simulink model "sig_kadet"  (R2022a)
settings: Solver=FixedStepAuto  StartTime=0.0  StopTime=10.0  FixedStep=framePeriod_s  RelTol=1e-3
undefined symbols (not defined in the file): Control, DiscIntNeverNeededParam, framePeriod_s
libraries: slpidlib x10, aerolibconvert2 x7, simulink_extras x2
(part 2 of 2)

== system sig_kadet/Control Laws/Attitude Feedback/Pitch Controller ==
  note: Pitch damper
  note: Map stick to pitch angle command
  Pitch Stick : Inport
  Pitch Angle [rad] : Inport  Port=2
  Pitch Rate [rad/s] : Inport  Port=3
  Angle Conversion : aerolibconvert2/Angle Conversion  IU=deg  OU=rad
  Constant : Constant  Value=Control.Attitude.Pitch.ref_deg  OutDataTypeStr=single
  Constant1 : Constant  Value=Control.Attitude.Pitch.d  OutDataTypeStr=single
  Constant2 : Constant  Value=framePeriod_s  OutDataTypeStr=single
  PID Controller : slpidlib/PID Controller  Controller=PID  Form=Parallel  TimeDomain=Discrete-time  UseExternalTs=on  SampleTime=-1  IntegratorMethod=Forward Euler  FilterMethod=Forward Euler  ControllerParametersSource=internal  P=Control.Attitude.Pitch.p  I=Control.Attitude.Pitch.i  D=0  UseFilter=off  N=100  TunerSelectOption=Transfer Function Based (PID Tuner App)  ZeroCross=off  InitialConditionSource=internal  InitialConditionForIntegrator=0  InitialConditionForFilter=0  DifferentiatorICPrevScaledInput=0  ExternalReset=none  TrackingMode=off  Kt=1  LimitOutput=on  SatLimitsSource=internal  UpperSaturationLimit=deg2rad(Control.elev_lim_deg)  LowerSaturationLimit=-deg2rad(Control.elev_lim_deg)  LinearizeAsGain=on  AntiWindupMode=clamping  Kb=1  PGainOutDataTypeStr=single  PProdOutDataTypeStr=single  POutMin=[]  POutMax=[]  IGainOutDataTypeStr=single  IProdOutDataTypeStr=single  IOutMin=[]  IOutMax=[]  DGainOutDataTypeStr=single  DProdOutDataTypeStr=single  DOutMin=[]  DOutMax=[]  NOutMin=[]  NOutMax=[]  SumOutDataTypeStr=single  SumOutMin=[]  SumOutMax=[]  SaturationOutDataTypeStr=single  SaturationOutMin=[]  SaturationOutMax=[]  PParamMin=[]  PParamMax=[]  IParamMin=[]  IParamMax=[]  DParamMin=[]  DParamMax=[]  NParamMin=[]  NParamMax=[]  KbParamMin=[]  KbParamMax=[]  KtParamMin=[]  KtParamMax=[]  KbOutMin=[]  KbOutMax=[]  KtOutMin=[]  KtOutMax=[]  IntegratorOutMin=[]  IntegratorOutMax=[]  FilterOutMin=[]  FilterOutMax=[]  SumI1OutMin=[]  SumI1OutMax=[]  SumI2OutMin=[]  SumI2OutMax=[]  SumI3OutMin=[]  SumI3OutMax=[]  SumI4OutMin=[]  SumI4OutMax=[]  SumDOutMin=[]  SumDOutMax=[]  DifferentiatorOutMin=[]  DifferentiatorOutMax=[]  FilterDiffOutCoefMin=[]  FilterDiffOutCoefMax=[]  ReciprocalOutMin=[]  ReciprocalOutMax=[]  SumDenOutMin=[]  SumDenOutMax=[]  SumNumOutMin=[]  SumNumOutMax=[]  DivideOutMin=[]  DivideOutMax=[]  UdiffTsProdOutMin=[]  UdiffTsProdOutMax=[]  NTsProdOutMin=[]  NTsProdOutMax=[]  UintegralTsProdOutMin=[]  UintegralTsProdOutMax=[]  UngainTsProdOutMin=[]  UngainTsProdOutMax=[]  IntegratorContinuousStateAttributes=''  IntegratorStateMustResolveToSignalObject=off  IntegratorRTWStateStorageClass=Auto  FilterContinuousStateAttributes=''  FilterStateMustResolveToSignalObject=off  FilterRTWStateStorageClass=Auto  ParallelPVariant=InternalParameters  IdealPVariant=Disabled  IVariant=InternalParameters  DVariant=InternalParameters  IntegratorVariant=Discrete  SatVariant=Enabled  AWVariant=DiscClampingParallel  PCopyVariant=Disabled  TRVariant=Disabled  FdbkBlocksVariant=Forward  IdealPFdbkVariant=Disabled  SatFdbkVariant=Disabled  DerivativeFilterVariant=Differentiator  NVariant=Passthrough  NCopyVariant=Disabled_SignalSpec  FilterICVariant=InternalICsDifferentiator  IntegratorICVariant=InternalICs  ExternalResetVariant=Disabled  TRSumVariant=Passthrough  SumFdbkVariant=Disabled  SumVariant=Sum_PID  TsampFilterVariant=ExternalTs  TsampNgainVariant=Passthrough  TsampIntegralVariant=ExternalTs  ExternalSaturationOutDataTypeStr=Inherit: Same as second input
  Product : Product  OutDataTypeStr=single
  Product1 : Product
  Subtract : Sum  Inputs=+-
  Subtract1 : Sum  Inputs=+-
  Elevator Cmd [rad] : Outport
  wires:
  Pitch Stick/1 -> Product/2
  Constant/1 -> Product/1
  Product/1 -> Angle Conversion/1
  Angle Conversion/1 -> Subtract/1
  Pitch Angle [rad]/1 -> Subtract/2
  PID Controller/1 -> Subtract1/1
  Product1/1 -> Subtract1/2
  Pitch Rate [rad/s]/1 -> Product1/1
  Constant1/1 -> Product1/2
  Subtract1/1 -> Elevator Cmd [rad]/1
  Constant2/1 -> PID Controller/2
  Subtract/1 -> PID Controller/1

== system sig_kadet/Control Laws/Attitude Feedback/Roll Controller ==
  note: Map stick to roll angle command
  note: Roll damper
  Roll Stick : Inport
  Roll Angle [rad] : Inport  Port=2
  Roll Rate [rad/s] : Inport  Port=3
  Angle Conversion : aerolibconvert2/Angle Conversion  IU=deg  OU=rad
  Constant : Constant  Value=Control.Attitude.Roll.ref_deg  OutDataTypeStr=single
  Constant1 : Constant  Value=Control.Attitude.Roll.d  OutDataTypeStr=single
  Constant2 : Constant  Value=framePeriod_s  OutDataTypeStr=single
  PID Controller : slpidlib/PID Controller  Controller=PID  Form=Parallel  TimeDomain=Discrete-time  UseExternalTs=on  SampleTime=-1  IntegratorMethod=Forward Euler  FilterMethod=Forward Euler  ControllerParametersSource=internal  P=Control.Attitude.Roll.p  I=Control.Attitude.Roll.i  D=0  UseFilter=off  N=100  TunerSelectOption=Transfer Function Based (PID Tuner App)  ZeroCross=off  InitialConditionSource=internal  InitialConditionForIntegrator=0  InitialConditionForFilter=0  DifferentiatorICPrevScaledInput=0  ExternalReset=none  TrackingMode=off  Kt=1  LimitOutput=on  SatLimitsSource=internal  UpperSaturationLimit=deg2rad(Control.ail_lim_deg)  LowerSaturationLimit=-deg2rad(Control.ail_lim_deg)  LinearizeAsGain=on  AntiWindupMode=clamping  Kb=1  PGainOutDataTypeStr=single  PProdOutDataTypeStr=single  POutMin=[]  POutMax=[]  IGainOutDataTypeStr=single  IProdOutDataTypeStr=single  IOutMin=[]  IOutMax=[]  DGainOutDataTypeStr=single  DProdOutDataTypeStr=single  DOutMin=[]  DOutMax=[]  NOutMin=[]  NOutMax=[]  SumOutDataTypeStr=single  SumOutMin=[]  SumOutMax=[]  SaturationOutDataTypeStr=single  SaturationOutMin=[]  SaturationOutMax=[]  PParamMin=[]  PParamMax=[]  IParamMin=[]  IParamMax=[]  DParamMin=[]  DParamMax=[]  NParamMin=[]  NParamMax=[]  KbParamMin=[]  KbParamMax=[]  KtParamMin=[]  KtParamMax=[]  KbOutMin=[]  KbOutMax=[]  KtOutMin=[]  KtOutMax=[]  IntegratorOutMin=[]  IntegratorOutMax=[]  FilterOutMin=[]  FilterOutMax=[]  SumI1OutMin=[]  SumI1OutMax=[]  SumI2OutMin=[]  SumI2OutMax=[]  SumI3OutMin=[]  SumI3OutMax=[]  SumI4OutMin=[]  SumI4OutMax=[]  SumDOutMin=[]  SumDOutMax=[]  DifferentiatorOutMin=[]  DifferentiatorOutMax=[]  FilterDiffOutCoefMin=[]  FilterDiffOutCoefMax=[]  ReciprocalOutMin=[]  ReciprocalOutMax=[]  SumDenOutMin=[]  SumDenOutMax=[]  SumNumOutMin=[]  SumNumOutMax=[]  DivideOutMin=[]  DivideOutMax=[]  UdiffTsProdOutMin=[]  UdiffTsProdOutMax=[]  NTsProdOutMin=[]  NTsProdOutMax=[]  UintegralTsProdOutMin=[]  UintegralTsProdOutMax=[]  UngainTsProdOutMin=[]  UngainTsProdOutMax=[]  IntegratorContinuousStateAttributes=''  IntegratorStateMustResolveToSignalObject=off  IntegratorRTWStateStorageClass=Auto  FilterContinuousStateAttributes=''  FilterStateMustResolveToSignalObject=off  FilterRTWStateStorageClass=Auto  ParallelPVariant=InternalParameters  IdealPVariant=Disabled  IVariant=InternalParameters  DVariant=InternalParameters  IntegratorVariant=Discrete  SatVariant=Enabled  AWVariant=DiscClampingParallel  PCopyVariant=Disabled  TRVariant=Disabled  FdbkBlocksVariant=Forward  IdealPFdbkVariant=Disabled  SatFdbkVariant=Disabled  DerivativeFilterVariant=Differentiator  NVariant=Passthrough  NCopyVariant=Disabled_SignalSpec  FilterICVariant=InternalICsDifferentiator  IntegratorICVariant=InternalICs  ExternalResetVariant=Disabled  TRSumVariant=Passthrough  SumFdbkVariant=Disabled  SumVariant=Sum_PID  TsampFilterVariant=ExternalTs  TsampNgainVariant=Passthrough  TsampIntegralVariant=ExternalTs  ExternalSaturationOutDataTypeStr=Inherit: Same as second input
  Product : Product  OutDataTypeStr=single
  Product1 : Product
  Subtract : Sum  Inputs=+-
  Subtract1 : Sum  Inputs=+-
  Aileron Cmd [rad] : Outport
  wires:
  Constant2/1 -> PID Controller/2
  Subtract1/1 -> Aileron Cmd [rad]/1
  Constant1/1 -> Product1/2
  Roll Rate [rad/s]/1 -> Product1/1
  Product1/1 -> Subtract1/2
  PID Controller/1 -> Subtract1/1
  Subtract/1 -> PID Controller/1
  Roll Angle [rad]/1 -> Subtract/2
  Angle Conversion/1 -> Subtract/1
  Product/1 -> Angle Conversion/1
  Constant/1 -> Product/1
  Roll Stick/1 -> Product/2

== system sig_kadet/Control Laws/Attitude Feedback/Yaw Damper ==
  Yaw Rate [rad/s] : Inport
  Discrete Transfer Fcn : DiscreteTransferFcn  Numerator=[-0.065 0.065]  Denominator=[1 -0.9608]
  Rudder Cmd [rad] : Outport
  wires:
  Discrete Transfer Fcn/1 -> Rudder Cmd [rad]/1
  Yaw Rate [rad/s]/1 -> Discrete Transfer Fcn/1

== system sig_kadet/Control Laws/Autopilot/Geschwindigkeitsregler ==
  note: desired airspeed for current waypoint
  Vehicle States : Inport
  Telemetry Data : Inport  Port=2
  Bus Selector : BusSelector  OutputSignals=ias_mps
  Bus Selector1 : BusSelector  OutputSignals=param1
  Bus Selector2 : BusSelector  OutputSignals=flight_plan,current_waypoint
  PID Controller : slpidlib/PID Controller  Controller=PID  Form=Parallel  TimeDomain=Discrete-time  UseExternalTs=on  SampleTime=-1  IntegratorMethod=Forward Euler  FilterMethod=Forward Euler  ControllerParametersSource=internal  P=1  I=1  D=0  UseFilter=off  N=100  TunerSelectOption=Transfer Function Based (PID Tuner App)  InitialConditionSource=internal  InitialConditionForIntegrator=0  InitialConditionForFilter=0  DifferentiatorICPrevScaledInput=0  ExternalReset=none  TrackingMode=off  Kt=1  LimitOutput=off  SatLimitsSource=internal  UpperSaturationLimit=inf  LowerSaturationLimit=-inf  LinearizeAsGain=on  AntiWindupMode=none  Kb=1  POutMin=[]  POutMax=[]  IOutMin=[]  IOutMax=[]  DOutMin=[]  DOutMax=[]  NOutMin=[]  NOutMax=[]  SumOutMin=[]  SumOutMax=[]  SaturationOutMin=[]  SaturationOutMax=[]  PParamMin=[]  PParamMax=[]  IParamMin=[]  IParamMax=[]  DParamMin=[]  DParamMax=[]  NParamMin=[]  NParamMax=[]  KbParamMin=[]  KbParamMax=[]  KtParamMin=[]  KtParamMax=[]  KbOutMin=[]  KbOutMax=[]  KtOutMin=[]  KtOutMax=[]  IntegratorOutMin=[]  IntegratorOutMax=[]  FilterOutMin=[]  FilterOutMax=[]  SumI1OutMin=[]  SumI1OutMax=[]  SumI2OutMin=[]  SumI2OutMax=[]  SumI3OutMin=[]  SumI3OutMax=[]  SumI4OutMin=[]  SumI4OutMax=[]  SumDOutMin=[]  SumDOutMax=[]  DifferentiatorOutMin=[]  DifferentiatorOutMax=[]  FilterDiffOutCoefMin=[]  FilterDiffOutCoefMax=[]  ReciprocalOutMin=[]  ReciprocalOutMax=[]  SumDenOutMin=[]  SumDenOutMax=[]  SumNumOutMin=[]  SumNumOutMax=[]  DivideOutMin=[]  DivideOutMax=[]  UdiffTsProdOutMin=[]  UdiffTsProdOutMax=[]  NTsProdOutMin=[]  NTsProdOutMax=[]  UintegralTsProdOutMin=[]  UintegralTsProdOutMax=[]  UngainTsProdOutMin=[]  UngainTsProdOutMax=[]  IntegratorContinuousStateAttributes=''  IntegratorStateMustResolveToSignalObject=off  IntegratorRTWStateStorageClass=Auto  FilterContinuousStateAttributes=''  FilterStateMustResolveToSignalObject=off  FilterRTWStateStorageClass=Auto  ParallelPVariant=InternalParameters  IdealPVariant=Disabled  IVariant=InternalParameters  DVariant=InternalParameters  IntegratorVariant=Discrete  SatVariant=Disabled  AWVariant=Passthrough  PCopyVariant=Disabled  TRVariant=Disabled  FdbkBlocksVariant=Forward  IdealPFdbkVariant=Disabled  SatFdbkVariant=Disabled  DerivativeFilterVariant=Differentiator  NVariant=Passthrough  NCopyVariant=Disabled_SignalSpec  FilterICVariant=InternalICsDifferentiator  IntegratorICVariant=InternalICs  ExternalResetVariant=Disabled  TRSumVariant=Passthrough  SumFdbkVariant=Disabled  SumVariant=Sum_PID  TsampFilterVariant=ExternalTs  TsampNgainVariant=Passthrough  TsampIntegralVariant=ExternalTs  ExternalSaturationOutDataTypeStr=Inherit: Same as second input
  Selector : Selector  IndexMode=Zero-based  InputPortWidth=500  IndexOptions=Index vector (port)  Indices=[1 3]  OutputSizes=1
  Sum : Sum  Inputs=|+-
  Throttle [0-1] : Outport
  wires:
  Vehicle States/1 -> Bus Selector/1
  Bus Selector/1 -> Sum/2  "<ias_mps>"
  Telemetry Data/1 -> Bus Selector2/1
  Bus Selector2/1 -> Selector/1  "<flight_plan>"
  Selector/1 -> Bus Selector1/1  "current waypoint parameter"
  Bus Selector2/2 -> Selector/2  "<current_waypoint>"
  Bus Selector1/1 -> Sum/1  "<param1>"
  Sum/1 -> PID Controller/1  "airspeed error [m/s]"
  PID Controller/1 -> Throttle [0-1]/1  "Throttle [0-1]"

== system sig_kadet/Control Laws/Autopilot/Gierdämpfer ==
  Vehicle States : Inport
  Bus Selector : BusSelector  OutputSignals=gyro_radps
  Demux : Demux  Outputs=3
  Discrete Transfer Fcn : DiscreteTransferFcn  Denominator=[1 6]
  Gain : Gain
  Terminator : Terminator
  Terminator1 : Terminator
  Out1 : Outport
  wires:
  Vehicle States/1 -> Bus Selector/1
  Bus Selector/1 -> Demux/1  "<gyro_radps>"
  Demux/1 -> Terminator/1  "p [rad/s]"
  Demux/2 -> Terminator1/1  "q [rad/s]"
  Demux/3 -> Gain/1  "r [rad/s]"
  Gain/1 -> Discrete Transfer Fcn/1

== system sig_kadet/Control Laws/Autopilot/Headingregler ==
  x aircraft [m] : Inport
  y aircraft [m] : Inport  Port=2
  x waypoint [m] : Inport  Port=3
  y waypoint [m] : Inport  Port=4
  Vehicle States : Inport  Port=5
  Bus Selector : BusSelector  OutputSignals=heading_rad
  MATLAB Function : MATLAB Function  TreatAsAtomicUnit=on
  PID Controller : slpidlib/PID Controller  Controller=PID  Form=Parallel  TimeDomain=Discrete-time  UseExternalTs=on  SampleTime=-1  IntegratorMethod=Forward Euler  FilterMethod=Forward Euler  ControllerParametersSource=internal  P=1  I=0  D=0  UseFilter=off  N=100  TunerSelectOption=Transfer Function Based (PID Tuner App)  InitialConditionSource=internal  InitialConditionForIntegrator=0  InitialConditionForFilter=0  DifferentiatorICPrevScaledInput=0  ExternalReset=none  TrackingMode=off  Kt=1  LimitOutput=off  SatLimitsSource=internal  UpperSaturationLimit=inf  LowerSaturationLimit=-inf  LinearizeAsGain=on  AntiWindupMode=none  Kb=1  POutMin=[]  POutMax=[]  IOutMin=[]  IOutMax=[]  DOutMin=[]  DOutMax=[]  NOutMin=[]  NOutMax=[]  SumOutMin=[]  SumOutMax=[]  SaturationOutMin=[]  SaturationOutMax=[]  PParamMin=[]  PParamMax=[]  IParamMin=[]  IParamMax=[]  DParamMin=[]  DParamMax=[]  NParamMin=[]  NParamMax=[]  KbParamMin=[]  KbParamMax=[]  KtParamMin=[]  KtParamMax=[]  KbOutMin=[]  KbOutMax=[]  KtOutMin=[]  KtOutMax=[]  IntegratorOutMin=[]  IntegratorOutMax=[]  FilterOutMin=[]  FilterOutMax=[]  SumI1OutMin=[]  SumI1OutMax=[]  SumI2OutMin=[]  SumI2OutMax=[]  SumI3OutMin=[]  SumI3OutMax=[]  SumI4OutMin=[]  SumI4OutMax=[]  SumDOutMin=[]  SumDOutMax=[]  DifferentiatorOutMin=[]  DifferentiatorOutMax=[]  FilterDiffOutCoefMin=[]  FilterDiffOutCoefMax=[]  ReciprocalOutMin=[]  ReciprocalOutMax=[]  SumDenOutMin=[]  SumDenOutMax=[]  SumNumOutMin=[]  SumNumOutMax=[]  DivideOutMin=[]  DivideOutMax=[]  UdiffTsProdOutMin=[]  UdiffTsProdOutMax=[]  NTsProdOutMin=[]  NTsProdOutMax=[]  UintegralTsProdOutMin=[]  UintegralTsProdOutMax=[]  UngainTsProdOutMin=[]  UngainTsProdOutMax=[]  IntegratorContinuousStateAttributes=''  IntegratorStateMustResolveToSignalObject=off  IntegratorRTWStateStorageClass=Auto  FilterContinuousStateAttributes=''  FilterStateMustResolveToSignalObject=off  FilterRTWStateStorageClass=Auto  ParallelPVariant=InternalParameters  IdealPVariant=Disabled  IVariant=InternalParameters  DVariant=InternalParameters  IntegratorVariant=Discrete  SatVariant=Disabled  AWVariant=Passthrough  PCopyVariant=Disabled  TRVariant=Disabled  FdbkBlocksVariant=Forward  IdealPFdbkVariant=Disabled  SatFdbkVariant=Disabled  DerivativeFilterVariant=Differentiator  NVariant=Passthrough  NCopyVariant=Disabled_SignalSpec  FilterICVariant=InternalICsDifferentiator  IntegratorICVariant=InternalICs  ExternalResetVariant=Disabled  TRSumVariant=Passthrough  SumFdbkVariant=Disabled  SumVariant=Sum_PID  TsampFilterVariant=ExternalTs  TsampNgainVariant=Passthrough  TsampIntegralVariant=ExternalTs  ExternalSaturationOutDataTypeStr=Inherit: Same as second input
  aileronausschlag : Outport
  heading error : Outport  Port=2
  wires:
  x aircraft [m]/1 -> MATLAB Function/1(x_ac)
  y aircraft [m]/1 -> MATLAB Function/2(y_ac)
  x waypoint [m]/1 -> MATLAB Function/3(x_wp)
  y waypoint [m]/1 -> MATLAB Function/4(y_wp)
  Vehicle States/1 -> Bus Selector/1
  Bus Selector/1 -> MATLAB Function/5(heading)  "<heading_rad>"
  MATLAB Function/1(heading_error) -> heading error/1, PID Controller/1
  PID Controller/1 -> aileronausschlag/1  "aileron ausschlag"

== system sig_kadet/Control Laws/Autopilot/Höhenregler ==
  z_aircraft [m] : Inport
  z_waypoint [m] : Inport  Port=2
  Vehicel States : Inport  Port=3
  Bus Selector : BusSelector  OutputSignals=pitch_rad,gyro_radps
  Demux : Demux  Outputs=3
  PID Controller : slpidlib/PID Controller  Controller=PID  Form=Parallel  TimeDomain=Discrete-time  UseExternalTs=on  SampleTime=-1  IntegratorMethod=Forward Euler  FilterMethod=Forward Euler  ControllerParametersSource=internal  P=1  I=1  D=0  UseFilter=off  N=100  TunerSelectOption=Transfer Function Based (PID Tuner App)  InitialConditionSource=internal  InitialConditionForIntegrator=0  InitialConditionForFilter=0  DifferentiatorICPrevScaledInput=0  ExternalReset=none  TrackingMode=off  Kt=1  LimitOutput=off  SatLimitsSource=internal  UpperSaturationLimit=inf  LowerSaturationLimit=-inf  LinearizeAsGain=on  AntiWindupMode=none  Kb=1  POutMin=[]  POutMax=[]  IOutMin=[]  IOutMax=[]  DOutMin=[]  DOutMax=[]  NOutMin=[]  NOutMax=[]  SumOutMin=[]  SumOutMax=[]  SaturationOutMin=[]  SaturationOutMax=[]  PParamMin=[]  PParamMax=[]  IParamMin=[]  IParamMax=[]  DParamMin=[]  DParamMax=[]  NParamMin=[]  NParamMax=[]  KbParamMin=[]  KbParamMax=[]  KtParamMin=[]  KtParamMax=[]  KbOutMin=[]  KbOutMax=[]  KtOutMin=[]  KtOutMax=[]  IntegratorOutMin=[]  IntegratorOutMax=[]  FilterOutMin=[]  FilterOutMax=[]  SumI1OutMin=[]  SumI1OutMax=[]  SumI2OutMin=[]  SumI2OutMax=[]  SumI3OutMin=[]  SumI3OutMax=[]  SumI4OutMin=[]  SumI4OutMax=[]  SumDOutMin=[]  SumDOutMax=[]  DifferentiatorOutMin=[]  DifferentiatorOutMax=[]  FilterDiffOutCoefMin=[]  FilterDiffOutCoefMax=[]  ReciprocalOutMin=[]  ReciprocalOutMax=[]  SumDenOutMin=[]  SumDenOutMax=[]  SumNumOutMin=[]  SumNumOutMax=[]  DivideOutMin=[]  DivideOutMax=[]  UdiffTsProdOutMin=[]  UdiffTsProdOutMax=[]  NTsProdOutMin=[]  NTsProdOutMax=[]  UintegralTsProdOutMin=[]  UintegralTsProdOutMax=[]  UngainTsProdOutMin=[]  UngainTsProdOutMax=[]  IntegratorContinuousStateAttributes=''  IntegratorStateMustResolveToSignalObject=off  IntegratorRTWStateStorageClass=Auto  FilterContinuousStateAttributes=''  FilterStateMustResolveToSignalObject=off  FilterRTWStateStorageClass=Auto  ParallelPVariant=InternalParameters  IdealPVariant=Disabled  IVariant=InternalParameters  DVariant=InternalParameters  IntegratorVariant=Discrete  SatVariant=Disabled  AWVariant=Passthrough  PCopyVariant=Disabled  TRVariant=Disabled  FdbkBlocksVariant=Forward  IdealPFdbkVariant=Disabled  SatFdbkVariant=Disabled  DerivativeFilterVariant=Differentiator  NVariant=Passthrough  NCopyVariant=Disabled_SignalSpec  FilterICVariant=InternalICsDifferentiator  IntegratorICVariant=InternalICs  ExternalResetVariant=Disabled  TRSumVariant=Passthrough  SumFdbkVariant=Disabled  SumVariant=Sum_PID  TsampFilterVariant=ExternalTs  TsampNgainVariant=Passthrough  TsampIntegralVariant=ExternalTs  ExternalSaturationOutDataTypeStr=Inherit: Same as second input
  PID Controller1 : slpidlib/PID Controller  Controller=PID  Form=Parallel  TimeDomain=Discrete-time  UseExternalTs=on  SampleTime=-1  IntegratorMethod=Forward Euler  FilterMethod=Forward Euler  ControllerParametersSource=internal  P=1  I=1  D=0  UseFilter=off  N=100  TunerSelectOption=Transfer Function Based (PID Tuner App)  InitialConditionSource=internal  InitialConditionForIntegrator=0  InitialConditionForFilter=0  DifferentiatorICPrevScaledInput=0  ExternalReset=none  TrackingMode=off  Kt=1  LimitOutput=off  SatLimitsSource=internal  UpperSaturationLimit=inf  LowerSaturationLimit=-inf  LinearizeAsGain=on  AntiWindupMode=none  Kb=1  POutMin=[]  POutMax=[]  IOutMin=[]  IOutMax=[]  DOutMin=[]  DOutMax=[]  NOutMin=[]  NOutMax=[]  SumOutMin=[]  SumOutMax=[]  SaturationOutMin=[]  SaturationOutMax=[]  PParamMin=[]  PParamMax=[]  IParamMin=[]  IParamMax=[]  DParamMin=[]  DParamMax=[]  NParamMin=[]  NParamMax=[]  KbParamMin=[]  KbParamMax=[]  KtParamMin=[]  KtParamMax=[]  KbOutMin=[]  KbOutMax=[]  KtOutMin=[]  KtOutMax=[]  IntegratorOutMin=[]  IntegratorOutMax=[]  FilterOutMin=[]  FilterOutMax=[]  SumI1OutMin=[]  SumI1OutMax=[]  SumI2OutMin=[]  SumI2OutMax=[]  SumI3OutMin=[]  SumI3OutMax=[]  SumI4OutMin=[]  SumI4OutMax=[]  SumDOutMin=[]  SumDOutMax=[]  DifferentiatorOutMin=[]  DifferentiatorOutMax=[]  FilterDiffOutCoefMin=[]  FilterDiffOutCoefMax=[]  ReciprocalOutMin=[]  ReciprocalOutMax=[]  SumDenOutMin=[]  SumDenOutMax=[]  SumNumOutMin=[]  SumNumOutMax=[]  DivideOutMin=[]  DivideOutMax=[]  UdiffTsProdOutMin=[]  UdiffTsProdOutMax=[]  NTsProdOutMin=[]  NTsProdOutMax=[]  UintegralTsProdOutMin=[]  UintegralTsProdOutMax=[]  UngainTsProdOutMin=[]  UngainTsProdOutMax=[]  IntegratorContinuousStateAttributes=''  IntegratorStateMustResolveToSignalObject=off  IntegratorRTWStateStorageClass=Auto  FilterContinuousStateAttributes=''  FilterStateMustResolveToSignalObject=off  FilterRTWStateStorageClass=Auto  ParallelPVariant=InternalParameters  IdealPVariant=Disabled  IVariant=InternalParameters  DVariant=InternalParameters  IntegratorVariant=Discrete  SatVariant=Disabled  AWVariant=Passthrough  PCopyVariant=Disabled  TRVariant=Disabled  FdbkBlocksVariant=Forward  IdealPFdbkVariant=Disabled  SatFdbkVariant=Disabled  DerivativeFilterVariant=Differentiator  NVariant=Passthrough  NCopyVariant=Disabled_SignalSpec  FilterICVariant=InternalICsDifferentiator  IntegratorICVariant=InternalICs  ExternalResetVariant=Disabled  TRSumVariant=Passthrough  SumFdbkVariant=Disabled  SumVariant=Sum_PID  TsampFilterVariant=ExternalTs  TsampNgainVariant=Passthrough  TsampIntegralVariant=ExternalTs  ExternalSaturationOutDataTypeStr=Inherit: Same as second input
  Sum : Sum  Inputs=|+-
  Sum1 : Sum  Inputs=|+-
  Sum2 : Sum  Inputs=|+-
  Terminator : Terminator
  Terminator1 : Terminator
  pitchrate damping gain : Gain
  delta_eta [deg] : Outport
  wires:
  z_waypoint [m]/1 -> Sum/1
  z_aircraft [m]/1 -> Sum/2
  Sum/1 -> PID Controller/1  "delta_z [m]"
  Vehicel States/1 -> Bus Selector/1
  Bus Selector/1 -> Sum1/2  "<pitch_rad>"
  PID Controller/1 -> Sum1/1  "desired pitch angele to get to desired altitude [rad]"
  Sum1/1 -> PID Controller1/1  "pitch angel error [rad]"
  PID Controller1/1 -> Sum2/1  "desired elevator deflection to get to desired pitch angle [deg]"
  Bus Selector/2 -> Demux/1  "<gyro_radps>"
  Demux/1 -> Terminator/1  "p [rad/s]"
  Demux/2 -> pitchrate damping gain/1  "q [rad/s]"
  Demux/3 -> Terminator1/1  "r [rad/s]"
  pitchrate damping gain/1 -> Sum2/2
  Sum2/1 -> delta_eta [deg]/1  "elevator deflection [deg]"

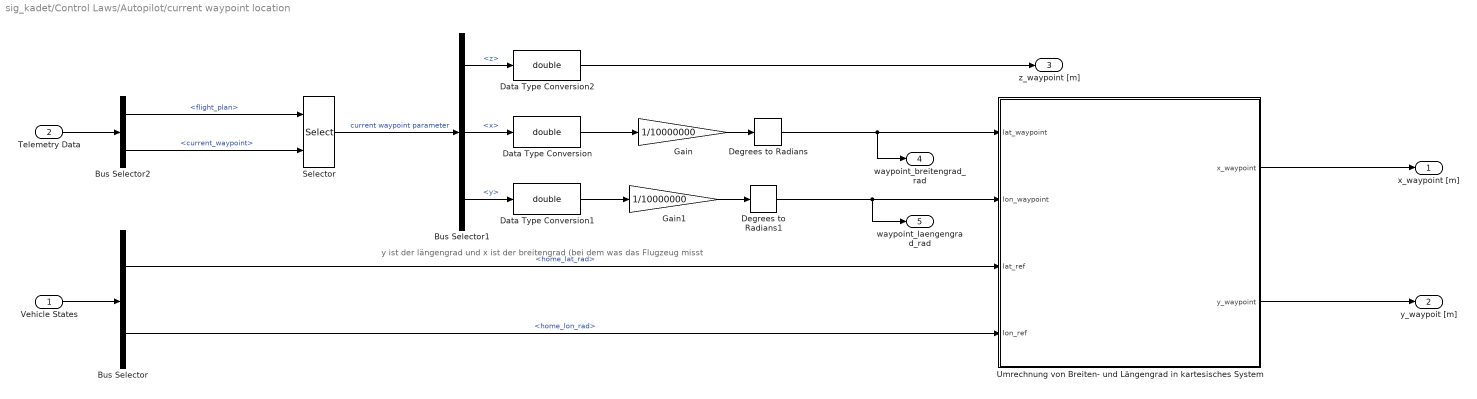
== system sig_kadet/Control Laws/Autopilot/current waypoint location ==
  note: y ist der längengrad und x ist der breitengrad (bei dem was das Flugzeug misst
  Vehicle States : Inport
  Telemetry Data : Inport  Port=2
  Bus Selector : BusSelector  OutputSignals=home_lat_rad,home_lon_rad
  Bus Selector1 : BusSelector  OutputSignals=z,x,y
  Bus Selector2 : BusSelector  OutputSignals=flight_plan,current_waypoint
  Data Type Conversion : DataTypeConversion  OutDataTypeStr=double  SaturateOnIntegerOverflow=off  RndMeth=Floor
  Data Type Conversion1 : DataTypeConversion  OutDataTypeStr=double  SaturateOnIntegerOverflow=off  RndMeth=Floor
  Data Type Conversion2 : DataTypeConversion  OutDataTypeStr=double  SaturateOnIntegerOverflow=off  RndMeth=Floor
  Degrees to Radians : simulink_extras/Transformations/Degrees to Radians
  Degrees to Radians1 : simulink_extras/Transformations/Degrees to Radians
  Gain : Gain  Gain=1/10000000
  Gain1 : Gain  Gain=1/10000000
  Selector : Selector  IndexMode=Zero-based  InputPortWidth=500  IndexOptions=Index vector (port)  Indices=[1 3]  OutputSizes=1
  Umrechnung von Breiten- und Längengrad in kartesisches System : MATLAB Function  TreatAsAtomicUnit=on
  x_waypoint [m] : Outport
  y_waypoit [m] : Outport  Port=2
  z_waypoint [m] : Outport  Port=3
  waypoint_breitengrad_rad : Outport  Port=4
  waypoint_laengengrad_rad : Outport  Port=5
  wires:
  Vehicle States/1 -> Bus Selector/1
  Telemetry Data/1 -> Bus Selector2/1
  Bus Selector2/1 -> Selector/1  "<flight_plan>"
  Bus Selector2/2 -> Selector/2  "<current_waypoint>"
  Selector/1 -> Bus Selector1/1  "current waypoint parameter"
  Bus Selector1/3 -> Data Type Conversion1/1  "<y>"
  Bus Selector1/2 -> Data Type Conversion/1  "<x>"
  Bus Selector1/1 -> Data Type Conversion2/1  "<z>"
  Bus Selector/1 -> Umrechnung von Breiten- und Längengrad in kartesisches System/3(lat_ref)  "<home_lat_rad>"
  Bus Selector/2 -> Umrechnung von Breiten- und Längengrad in kartesisches System/4(lon_ref)  "<home_lon_rad>"
  Umrechnung von Breiten- und Längengrad in kartesisches System/1(x_waypoint) -> x_waypoint [m]/1
  Umrechnung von Breiten- und Längengrad in kartesisches System/2(y_waypoint) -> y_waypoit [m]/1
  Data Type Conversion/1 -> Gain/1
  Data Type Conversion1/1 -> Gain1/1
  Data Type Conversion2/1 -> z_waypoint [m]/1
  Gain/1 -> Degrees to Radians/1
  Degrees to Radians/1 -> Umrechnung von Breiten- und Längengrad in kartesisches System/1(lat_waypoint), waypoint_breitengrad_rad/1
  Gain1/1 -> Degrees to Radians1/1
  Degrees to Radians1/1 -> Umrechnung von Breiten- und Längengrad in kartesisches System/2(lon_waypoint), waypoint_laengengrad_rad/1

== system sig_kadet/Control Laws/Autopilot/plane location ==
  Vehicle States : Inport
  Bus Selector : BusSelector  OutputSignals=lat_rad,lon_rad,home_lat_rad,home_lon_rad,alt_msl_m
  Umrechnung von Breiten- und Längengrad in kartesisches System : MATLAB Function  TreatAsAtomicUnit=on
  x_aircraft [m] : Outport
  y_aircraft [m] : Outport  Port=2
  z_aircraft [m] : Outport  Port=3
  wires:
  Vehicle States/1 -> Bus Selector/1
  Bus Selector/2 -> Umrechnung von Breiten- und Längengrad in kartesisches System/2(lon_aircraft)  "<lon_rad>"
  Bus Selector/4 -> Umrechnung von Breiten- und Längengrad in kartesisches System/4(lon_ref)  "<home_lon_rad>"
  Bus Selector/1 -> Umrechnung von Breiten- und Längengrad in kartesisches System/1(lat_aircraft)  "<lat_rad>"
  Bus Selector/3 -> Umrechnung von Breiten- und Längengrad in kartesisches System/3(lat_ref)  "<home_lat_rad>"
  Bus Selector/5 -> z_aircraft [m]/1  "<alt_msl_m>"
  Umrechnung von Breiten- und Längengrad in kartesisches System/2(y_aircraft) -> y_aircraft [m]/1
  Umrechnung von Breiten- und Längengrad in kartesisches System/1(x_aircraft) -> x_aircraft [m]/1

== system sig_kadet/Control Laws/Autopilot/waypoint rached ==
  x_aircraft [m] : Inport
  y_aircraft [m] : Inport  Port=2
  x_waypoint [m] : Inport  Port=3
  y_waypoit [m] : Inport  Port=4
  Constant : Constant
  Constant1 : Constant  Value=0
  Data Type Conversion : DataTypeConversion  OutDataTypeStr=boolean  SaturateOnIntegerOverflow=off  RndMeth=Floor
  MATLAB Function : MATLAB Function  TreatAsAtomicUnit=on
  Switch : Switch  Criteria=u2 > Threshold  Threshold=10  SaturateOnIntegerOverflow=off  InputSameDT=off
  waypoint reached : Outport
  distance to waypoint [m] : Outport  Port=2
  wires:
  x_aircraft [m]/1 -> MATLAB Function/1(x_aircraft)
  y_aircraft [m]/1 -> MATLAB Function/2(y_aircraft)
  x_waypoint [m]/1 -> MATLAB Function/3(x_waypoint)
  y_waypoit [m]/1 -> MATLAB Function/4(y_waypoint)
  MATLAB Function/1(distance) -> distance to waypoint [m]/1, Switch/2  "distance to waypoint [m]"
  Switch/1 -> Data Type Conversion/1
  Constant/1 -> Switch/3
  Constant1/1 -> Switch/1
  Data Type Conversion/1 -> waypoint reached/1

== system sig_kadet/Control Laws/Altitude Hold/Attitude Feedback/Pitch Controller ==
  note: Pitch damper
  note: Map stick to pitch angle command
  Pitch Stick : Inport
  Pitch Angle [rad] : Inport  Port=2
  Pitch Rate [rad/s] : Inport  Port=3
  Angle Conversion : aerolibconvert2/Angle Conversion  IU=deg  OU=rad
  Constant : Constant  Value=Control.Attitude.Pitch.ref_deg  OutDataTypeStr=single
  Constant1 : Constant  Value=Control.Attitude.Pitch.d  OutDataTypeStr=single
  Constant2 : Constant  Value=framePeriod_s  OutDataTypeStr=single
  PID Controller : slpidlib/PID Controller  Controller=PID  Form=Parallel  TimeDomain=Discrete-time  UseExternalTs=on  SampleTime=-1  IntegratorMethod=Forward Euler  FilterMethod=Forward Euler  ControllerParametersSource=internal  P=Control.Attitude.Pitch.p  I=Control.Attitude.Pitch.i  D=0  UseFilter=off  N=100  TunerSelectOption=Transfer Function Based (PID Tuner App)  ZeroCross=off  InitialConditionSource=internal  InitialConditionForIntegrator=0  InitialConditionForFilter=0  DifferentiatorICPrevScaledInput=0  ExternalReset=none  TrackingMode=off  Kt=1  LimitOutput=on  SatLimitsSource=internal  UpperSaturationLimit=deg2rad(Control.elev_lim_deg)  LowerSaturationLimit=-deg2rad(Control.elev_lim_deg)  LinearizeAsGain=on  AntiWindupMode=clamping  Kb=1  PGainOutDataTypeStr=single  PProdOutDataTypeStr=single  POutMin=[]  POutMax=[]  IGainOutDataTypeStr=single  IProdOutDataTypeStr=single  IOutMin=[]  IOutMax=[]  DGainOutDataTypeStr=single  DProdOutDataTypeStr=single  DOutMin=[]  DOutMax=[]  NOutMin=[]  NOutMax=[]  SumOutDataTypeStr=single  SumOutMin=[]  SumOutMax=[]  SaturationOutDataTypeStr=single  SaturationOutMin=[]  SaturationOutMax=[]  PParamMin=[]  PParamMax=[]  IParamMin=[]  IParamMax=[]  DParamMin=[]  DParamMax=[]  NParamMin=[]  NParamMax=[]  KbParamMin=[]  KbParamMax=[]  KtParamMin=[]  KtParamMax=[]  KbOutMin=[]  KbOutMax=[]  KtOutMin=[]  KtOutMax=[]  IntegratorOutMin=[]  IntegratorOutMax=[]  FilterOutMin=[]  FilterOutMax=[]  SumI1OutMin=[]  SumI1OutMax=[]  SumI2OutMin=[]  SumI2OutMax=[]  SumI3OutMin=[]  SumI3OutMax=[]  SumI4OutMin=[]  SumI4OutMax=[]  SumDOutMin=[]  SumDOutMax=[]  DifferentiatorOutMin=[]  DifferentiatorOutMax=[]  FilterDiffOutCoefMin=[]  FilterDiffOutCoefMax=[]  ReciprocalOutMin=[]  ReciprocalOutMax=[]  SumDenOutMin=[]  SumDenOutMax=[]  SumNumOutMin=[]  SumNumOutMax=[]  DivideOutMin=[]  DivideOutMax=[]  UdiffTsProdOutMin=[]  UdiffTsProdOutMax=[]  NTsProdOutMin=[]  NTsProdOutMax=[]  UintegralTsProdOutMin=[]  UintegralTsProdOutMax=[]  UngainTsProdOutMin=[]  UngainTsProdOutMax=[]  IntegratorContinuousStateAttributes=''  IntegratorStateMustResolveToSignalObject=off  IntegratorRTWStateStorageClass=Auto  FilterContinuousStateAttributes=''  FilterStateMustResolveToSignalObject=off  FilterRTWStateStorageClass=Auto  ParallelPVariant=InternalParameters  IdealPVariant=Disabled  IVariant=InternalParameters  DVariant=InternalParameters  IntegratorVariant=Discrete  SatVariant=Enabled  AWVariant=DiscClampingParallel  PCopyVariant=Disabled  TRVariant=Disabled  FdbkBlocksVariant=Forward  IdealPFdbkVariant=Disabled  SatFdbkVariant=Disabled  DerivativeFilterVariant=Differentiator  NVariant=Passthrough  NCopyVariant=Disabled_SignalSpec  FilterICVariant=InternalICsDifferentiator  IntegratorICVariant=InternalICs  ExternalResetVariant=Disabled  TRSumVariant=Passthrough  SumFdbkVariant=Disabled  SumVariant=Sum_PID  TsampFilterVariant=ExternalTs  TsampNgainVariant=Passthrough  TsampIntegralVariant=ExternalTs  ExternalSaturationOutDataTypeStr=Inherit: Same as second input
  Product : Product  OutDataTypeStr=single
  Product1 : Product
  Subtract : Sum  Inputs=+-
  Subtract1 : Sum  Inputs=+-
  Elevator Cmd [rad] : Outport
  wires:
  Pitch Stick/1 -> Product/2
  Constant/1 -> Product/1
  Product/1 -> Angle Conversion/1
  Angle Conversion/1 -> Subtract/1
  Pitch Angle [rad]/1 -> Subtract/2
  Subtract/1 -> PID Controller/1
  PID Controller/1 -> Subtract1/1
  Product1/1 -> Subtract1/2
  Pitch Rate [rad/s]/1 -> Product1/1
  Constant1/1 -> Product1/2
  Subtract1/1 -> Elevator Cmd [rad]/1
  Constant2/1 -> PID Controller/2

== system sig_kadet/Control Laws/Altitude Hold/Attitude Feedback/Roll Controller ==
  note: Map stick to roll angle command
  note: Roll damper
  Roll Stick : Inport
  Roll Angle [rad] : Inport  Port=2
  Roll Rate [rad/s] : Inport  Port=3
  Angle Conversion : aerolibconvert2/Angle Conversion  IU=deg  OU=rad
  Constant : Constant  Value=Control.Attitude.Roll.ref_deg  OutDataTypeStr=single
  Constant1 : Constant  Value=Control.Attitude.Roll.d  OutDataTypeStr=single
  Constant2 : Constant  Value=framePeriod_s  OutDataTypeStr=single
  PID Controller : slpidlib/PID Controller  Controller=PID  Form=Parallel  TimeDomain=Discrete-time  UseExternalTs=on  SampleTime=-1  IntegratorMethod=Forward Euler  FilterMethod=Forward Euler  ControllerParametersSource=internal  P=Control.Attitude.Roll.p  I=Control.Attitude.Roll.i  D=0  UseFilter=off  N=100  TunerSelectOption=Transfer Function Based (PID Tuner App)  ZeroCross=off  InitialConditionSource=internal  InitialConditionForIntegrator=0  InitialConditionForFilter=0  DifferentiatorICPrevScaledInput=0  ExternalReset=none  TrackingMode=off  Kt=1  LimitOutput=on  SatLimitsSource=internal  UpperSaturationLimit=deg2rad(Control.ail_lim_deg)  LowerSaturationLimit=-deg2rad(Control.ail_lim_deg)  LinearizeAsGain=on  AntiWindupMode=clamping  Kb=1  PGainOutDataTypeStr=single  PProdOutDataTypeStr=single  POutMin=[]  POutMax=[]  IGainOutDataTypeStr=single  IProdOutDataTypeStr=single  IOutMin=[]  IOutMax=[]  DGainOutDataTypeStr=single  DProdOutDataTypeStr=single  DOutMin=[]  DOutMax=[]  NOutMin=[]  NOutMax=[]  SumOutDataTypeStr=single  SumOutMin=[]  SumOutMax=[]  SaturationOutDataTypeStr=single  SaturationOutMin=[]  SaturationOutMax=[]  PParamMin=[]  PParamMax=[]  IParamMin=[]  IParamMax=[]  DParamMin=[]  DParamMax=[]  NParamMin=[]  NParamMax=[]  KbParamMin=[]  KbParamMax=[]  KtParamMin=[]  KtParamMax=[]  KbOutMin=[]  KbOutMax=[]  KtOutMin=[]  KtOutMax=[]  IntegratorOutMin=[]  IntegratorOutMax=[]  FilterOutMin=[]  FilterOutMax=[]  SumI1OutMin=[]  SumI1OutMax=[]  SumI2OutMin=[]  SumI2OutMax=[]  SumI3OutMin=[]  SumI3OutMax=[]  SumI4OutMin=[]  SumI4OutMax=[]  SumDOutMin=[]  SumDOutMax=[]  DifferentiatorOutMin=[]  DifferentiatorOutMax=[]  FilterDiffOutCoefMin=[]  FilterDiffOutCoefMax=[]  ReciprocalOutMin=[]  ReciprocalOutMax=[]  SumDenOutMin=[]  SumDenOutMax=[]  SumNumOutMin=[]  SumNumOutMax=[]  DivideOutMin=[]  DivideOutMax=[]  UdiffTsProdOutMin=[]  UdiffTsProdOutMax=[]  NTsProdOutMin=[]  NTsProdOutMax=[]  UintegralTsProdOutMin=[]  UintegralTsProdOutMax=[]  UngainTsProdOutMin=[]  UngainTsProdOutMax=[]  IntegratorContinuousStateAttributes=''  IntegratorStateMustResolveToSignalObject=off  IntegratorRTWStateStorageClass=Auto  FilterContinuousStateAttributes=''  FilterStateMustResolveToSignalObject=off  FilterRTWStateStorageClass=Auto  ParallelPVariant=InternalParameters  IdealPVariant=Disabled  IVariant=InternalParameters  DVariant=InternalParameters  IntegratorVariant=Discrete  SatVariant=Enabled  AWVariant=DiscClampingParallel  PCopyVariant=Disabled  TRVariant=Disabled  FdbkBlocksVariant=Forward  IdealPFdbkVariant=Disabled  SatFdbkVariant=Disabled  DerivativeFilterVariant=Differentiator  NVariant=Passthrough  NCopyVariant=Disabled_SignalSpec  FilterICVariant=InternalICsDifferentiator  IntegratorICVariant=InternalICs  ExternalResetVariant=Disabled  TRSumVariant=Passthrough  SumFdbkVariant=Disabled  SumVariant=Sum_PID  TsampFilterVariant=ExternalTs  TsampNgainVariant=Passthrough  TsampIntegralVariant=ExternalTs  ExternalSaturationOutDataTypeStr=Inherit: Same as second input
  Product : Product  OutDataTypeStr=single
  Product1 : Product
  Subtract : Sum  Inputs=+-
  Subtract1 : Sum  Inputs=+-
  Aileron Cmd [rad] : Outport
  wires:
  Constant2/1 -> PID Controller/2
  Subtract1/1 -> Aileron Cmd [rad]/1
  Constant1/1 -> Product1/2
  Roll Rate [rad/s]/1 -> Product1/1
  Product1/1 -> Subtract1/2
  PID Controller/1 -> Subtract1/1
  Subtract/1 -> PID Controller/1
  Roll Angle [rad]/1 -> Subtract/2
  Angle Conversion/1 -> Subtract/1
  Product/1 -> Angle Conversion/1
  Constant/1 -> Product/1
  Roll Stick/1 -> Product/2

== system sig_kadet/Control Laws/Altitude Hold/Attitude Feedback/Yaw Damper ==
  Yaw Rate [rad/s] : Inport
  Discrete Transfer Fcn : DiscreteTransferFcn  Numerator=[-0.065 0.065]  Denominator=[1 -0.9608]
  Rudder Cmd [rad] : Outport
  wires:
  Discrete Transfer Fcn/1 -> Rudder Cmd [rad]/1
  Yaw Rate [rad/s]/1 -> Discrete Transfer Fcn/1

== matlab function sig_kadet/Control Laws/Autopilot/current waypoint location/Umrechnung von Breiten- und Längengrad in kartesisches System ==
  data: lat_waypoint input double; lon_waypoint input double; lat_ref input double; lon_ref input double; x_waypoint output double; y_waypoint output double
function [x_waypoint, y_waypoint] = latlon2xy(lat_waypoint, lon_waypoint, lat_ref, lon_ref)

% Breitengradumrechung
% 2 Meridiane ergeben einen Längenkreis, weil ein Meridian ein Halbkreis ist
% Die Meridiane also alle Linien bei denen der Längengrad konstant ist
% besitzen hier im vereinfachten Modell alle den gleichen Umfang uL
% Quelle: https://de.wikipedia.org/wiki/Meridian_(Geographie)#:~:text=Die%20L%C3%A4nge%20eines%20Meridians%20betr%C3%A4gt,liegen%2C%20bezeichnet%20man%20als%20Abweitung.

uL = 2*20003.93; % [km]

% Daraus folgt wie viel ein Grad auf dem Meridian (also ein Breitengrad) in
% m entspricht
% Breitegrd in Grad to Länge in m

Bg2l = uL/360*1000;



% Längengradumrechnung
% Der Umfang eines Breitenkreises ist abhängig vom Breitengrad
% Als Grundlage der Berechnung dient der Äquatorrdius rE
% Quelle: https://de.wikipedia.org/wiki/Erdradius

Bg = lat_waypoint; % [°] Breitengrad an dem wir den Umfang bestimmen wollen
rE = 6378; %[km] Äquatorradius
rBk = rE*cos(Bg);
uBk = 2*rBk*pi;

% Daraus folgt wie viel ein Grad auf dem Breitenkreis in m entspricht
% Längengrad in Grad to Länge in m

Lg2l = uBk/360*1000;

x_waypoint = rad2deg(lon_waypoint-lon_ref)*Lg2l;
y_waypoint = rad2deg(lat_waypoint-lat_ref)*Bg2l;

== matlab function sig_kadet/Control Laws/Autopilot/plane location/Umrechnung von Breiten- und Längengrad in kartesisches System ==
  data: lat_aircraft input double; lon_aircraft input double; lat_ref input double; lon_ref input double; x_aircraft output double; y_aircraft output double
function [x_aircraft, y_aircraft] = latlon2xy(lat_aircraft, lon_aircraft, lat_ref, lon_ref)

% Breitengradumrechung
% 2 Meridiane ergeben einen Längenkreis, weil ein Meridian ein Halbkreis ist
% Die Meridiane also alle Linien bei denen der Längengrad konstant ist
% besitzen hier im vereinfachten Modell alle den gleichen Umfang uL
% Quelle: https://de.wikipedia.org/wiki/Meridian_(Geographie)#:~:text=Die%20L%C3%A4nge%20eines%20Meridians%20betr%C3%A4gt,liegen%2C%20bezeichnet%20man%20als%20Abweitung.

uL = 2*20003.93; % [km]

% Daraus folgt wie viel ein Grad auf dem Meridian (also ein Breitengrad) in
% m entspricht
% Breitegrd in Grad to Länge in m

Bg2l = uL/360*1000;



% Längengradumrechnung
% Der Umfang eines Breitenkreises ist abhängig vom Breitengrad
% Als Grundlage der Berechnung dient der Äquatorrdius rE
% Quelle: https://de.wikipedia.org/wiki/Erdradius

Bg = lat_aircraft; % [°] Breitengrad an dem wir den Umfang bestimmen wollen
rE = 6378; %[km] Äquatorradius
rBk = rE*cos(Bg);
uBk = 2*rBk*pi;

% Daraus folgt wie viel ein Grad auf dem Breitenkreis in m entspricht
% Längengrad in Grad to Länge in m

Lg2l = uBk/360*1000;

x_aircraft = rad2deg(lon_aircraft-lon_ref)*Lg2l;
y_aircraft = rad2deg(lat_aircraft-lat_ref)*Bg2l;

== matlab function sig_kadet/Control Laws/Autopilot/waypoint rached/MATLAB Function ==
  data: x_aircraft input; distance output; y_aircraft input; x_waypoint input; y_waypoint input
function distance = fcn(x_aircraft, y_aircraft, x_waypoint, y_waypoint)

distance = sqrt((x_aircraft-x_waypoint)^2 + (y_aircraft-y_waypoint)^2)

== matlab function sig_kadet/Control Laws/Autopilot/Headingregler/MATLAB Function ==
  data: x_ac input; heading_error output; y_ac input; x_wp input; y_wp input; heading input
function heading_error = fcn(x_ac, y_ac, x_wp, y_wp, heading)
% ac ist der Vektor vom Koordinatenursprung zum Flugzeug
% wp ist der Vektor vom Koordiantenurspung zum Wegpunkt
% d ist der Vektor vom Flugzueg zum Wegpunkt
% h ist der heading-Vektor des Flugzeugs
% heading_error ist der Winkel in rad zwischen h und d. ist der Wegpunkt
% auf der rechten Seite vom FLugzueg so ist heading_error < 0, ist der
% Wegpunkt auf der linken Seite vom Flugzueg so ist heading_error > 0.
% headingerror ist Element von [-pi, pi]
ac = [x_ac; y_ac];
wp = [x_wp; y_wp];
d = wp - ac;
h = [sin(heading); cos(heading)];

% über das Skalarprodukt lässt sich nur der Betrag von heading_error
% bestimmen
heading_error_betrag = acos(dot(h,d)/(norm(h)*norm(d)));

% über das Kreuzprodukt von h und d kann herausgefunden werden, ob sich wp
% links oder rechts vom Flugzeug befindet. Zeigt das Kreuzprodukt: h x d in positive
% z-Richtung so liegt der Wegpunkt links vom Flugzeug, zeigt es in negative
% z-Richtung so so liegt der Wegpunkt rechts vom Flugzeug. Die z-Komponente
% von h x d kann mit det([h, d]) bestimmt werden. liegen h und d parallel
% zueinander (also heading_error_betrag = 0 oder = 180) so wird die
% z-Komponente von h x d zu 0 und somit auch sign(det[h, d]), das führt zu
% Problemen wenn das heading_error_betrag = 180° beträgt weshlab die if Bedingung
% notwendig ist. Mit der if Bedingung wie sie hier definiert ist gibt es
% kein heading_error = -180° sondern nur +180° und -179.99999°

o = sign(det([h d]));

if heading_error_betrag > 90 && sign(det([h d])) == 0
    heading_error = heading_error_betrag;
else
heading_error = o*heading_error_betrag;
end
